simulink library "theta_2_alpha"  (R2014b)
settings: Solver=ode45  StartTime=0.0  StopTime=10.0  RelTol=1e-3
values from neighbouring files (symbols this model uses):
  d = 0.02    [ball.m]    (also in ball_and_beam.m = 0.04; draft.m; parameter.m = 0.04)
  h1 = 0.0    (= 0)    [ball.m]    (also in draft.m)
  k = 0.08    [ball.m]    (also in ball_and_beam.m = 0.12; draft.m)
  l = 0.4    [ball.m]    (also in ball_and_beam.m; draft.m)
settings Model: Creator=nghia  LastModifiedBy=Admin

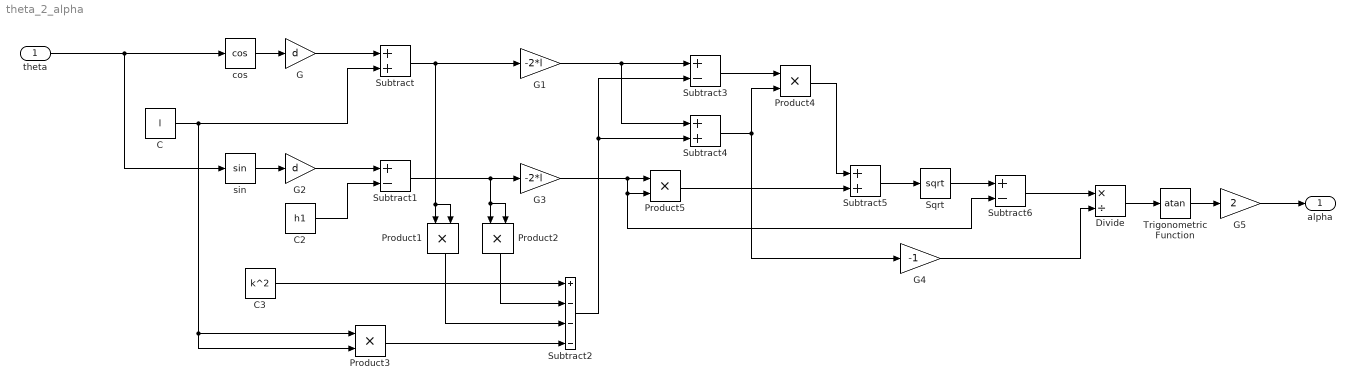
== system theta_2_alpha ==
  theta : Inport
  C : Constant  Value=l
  C2 : Constant  Value=h1
  C3 : Constant  Value=k^2
  Divide : Product  Inputs=*/
  G : Gain  Gain=d
  G1 : Gain  Gain=-2*l
  G2 : Gain  Gain=d
  G3 : Gain  Gain=-2*l
  G4 : Gain  Gain=-1
  G5 : Gain  Gain=2
  Product{1..5} (5 alike) : Product
  Sqrt : Sqrt  SaturateOnIntegerOverflow=on
  Subtract : Sum
  Subtract1 : Sum  Inputs=+-
  Subtract2 : Sum  Inputs=+---
  Subtract3 : Sum  Inputs=+-
  Subtract4 : Sum
  Subtract5 : Sum
  Subtract6 : Sum  Inputs=+-
  Trigonometric Function : Trigonometry  Operator=atan
  "cos " : Trigonometry  Operator=cos
  sin : Trigonometry
  alpha : Outport
  wires:
  Divide/1 -> Trigonometric Function/1
  G5/1 -> alpha/1
  theta/1 -> "cos "/1, sin/1
  Product2/1 -> Subtract2/2
  C3/1 -> Subtract2/1
  G4/1 -> Divide/2
  C/1 -> Product3/2, Product3/1, Subtract/2
  Subtract/1 -> Product1/2, Product1/1, G1/1
  "cos "/1 -> G/1
  Product1/1 -> Subtract2/3
  Subtract6/1 -> Divide/1
  G3/1 -> Subtract6/2, Product5/2, Product5/1
  Subtract5/1 -> Sqrt/1
  Subtract1/1 -> Product2/2, Product2/1, G3/1
  G2/1 -> Subtract1/1
  sin/1 -> G2/1
  C2/1 -> Subtract1/2
  Product5/1 -> Subtract5/2
  Subtract2/1 -> Subtract4/2, Subtract3/2
  Subtract3/1 -> Product4/1
  Trigonometric Function/1 -> G5/1
  Product4/1 -> Subtract5/1
  Sqrt/1 -> Subtract6/1
  Product3/1 -> Subtract2/4
  Subtract4/1 -> G4/1, Product4/2
  G1/1 -> Subtract3/1, Subtract4/1
  G/1 -> Subtract/1
